simulink model "mvc_model_L"  (R2019a)
settings: Solver=FixedStepAuto  StartTime=0.0  StopTime=500  FixedStep=Ts  RelTol=1e-3  EnableMultiTasking=on
values from neighbouring files (symbols this model uses):
  f1_off_L = 0    [msstudy.m]
  f2_off_L = 0    [msstudy.m]
  f3_off_L = 0    [msstudy.m]
  f4_off_L = 0    [msstudy.m]
  f5_off_L = 0    [msstudy.m]
  f6_off_L = 0    [msstudy.m]
  maxtorquediff = 50    [msstudy.m]
  off_TA = 0    [msstudy.m]    (also in mvc_reflex.m = nanmean(tsmovavg(Input3.data(1:20000,1),'s',1000,1)))
  TA_MVC = 1    [msstudy.m]    (also in mvc_reflex.m = max((tsmovavg(abs(Input3.data(:,1)-off_TA),'s',1000,1))))
  Ts = 0.0005    [msstudy.m]
  tweight = 50*0.01*weight    [msstudy.m]    (also in weightcalc.m = weight/2)
undefined symbols (not defined in the file or in its folder): Pull, up
libraries: speedgoatlib_IO183 x6, powerlib_meascontrol x3, slrtlib x2
settings Model: Creator=vnalam  LastModifiedBy=vnalam
settings DataIOCC: LimitDataPoints=on  SaveFormat=StructureWithTime  ReturnWorkspaceOutputs=off
settings OptimizationCC: BlockReduction=off  OptimizeBlockIOStorage=off  BufferReuse=off  GlobalBufferReuse=off  ExpressionFolding=off  LocalBlockOutputs=off  LifeSpan=inf  OptimizeDataStoreBuffers=off  BusAssignmentInplaceUpdate=off
settings DebuggingCC: AllowSymbolicDim=off  SFUnexpectedBacktrackingDiag=warning  SFNoUnconditionalDefaultTransitionDiag=warning  SFExecutionAtInitializationDiag=none  ArithmeticOperatorsInVariantConditions=warning
settings HardwareCC: ProdBitPerPointer=32  ProdBitPerSizeT=32  ProdBitPerPtrDiffT=32  ProdLargestAtomicFloat=None  ProdWordSize=32  ProdLongLongMode=on  ProdHWDeviceType=Generic->32-bit x86 compatible
settings ModelReferenceCC: PropagateSignalLabelsOutOfModel=off
settings SFSimCC: SimUseLocalCustomCode=off
settings RTWCC: SystemTargetFile=slrt.tlc  TLCOptions=-axPCModelStackSizeKB=512  TemplateMakefile=slrt_default_tmf  Description=Simulink Real-Time  RTWUseLocalCustomCode=off  CodeExecutionProfiling=on  RTWCompilerOptimization=on
settings CodeAppCC: StateflowObjectComments=on
settings SimulinkRealTimeCC: PreserveStateflowLocalDataDimensions=off  xPCisDownloadable=off
settings ConfigComp: CovMetricSettings=dw  CovHtmlReporting=on  CovSaveCumulativeToWorkspaceVar=on  CovSaveSingleToWorkspaceVar=on  CovExternalEMLEnable=off

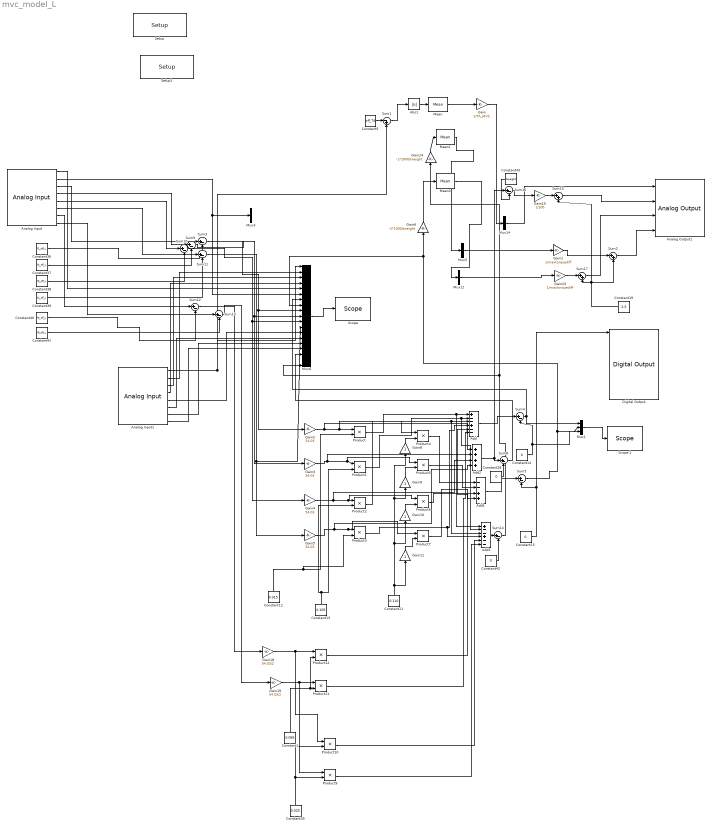
== system mvc_model_L ==
  Abs1 : Abs
  Add : Sum  Inputs=+--+--
  Add1 : Sum  Inputs=--++
  Add2 : Sum  Inputs=++++
  Add3 : Sum  Inputs=+--+--
  Analog Input : speedgoatlib_IO183/Analog Input  Priority=0  parModuleId=1  parSampTime=Ts  parPciSlot=-1  parAdChannelLow=1  parAdChannelHigh=8
      settings: SourceProductName=Simulink Real-Time: Speedgoat Library
  Analog Input1 : speedgoatlib_IO183/Analog Input  Priority=0  parModuleId=2  parSampTime=Ts  parPciSlot=-1  parAdChannelLow=1  parAdChannelHigh=8
      settings: SourceProductName=Simulink Real-Time: Speedgoat Library
  Analog Output1 : speedgoatlib_IO183/Analog Output  parModuleId=2  parSampTime=-1  parDaSimult=on  parPciSlot=-1  parDaChannels=[1 2 3 4]  parDaInit=[0 0 0 0]  parDaReset=[0 0 0 0]
      settings: SourceProductName=Simulink Real-Time: Speedgoat Library
  Constant1 : Constant  Value=0.095  SampleTime=-1
  Constant11 : Constant  Value=0.110  SampleTime=-1
  Constant12 : Constant  Value=0.315  SampleTime=-1
  Constant13 : Constant  Value=0.105  SampleTime=-1
  Constant{14..15,28,42} (4 alike) : Constant  Value=0  SampleTime=Ts
  Constant19 : Constant  Value=2.5  SampleTime=Ts
  Constant35 : Constant  Value=0.025  SampleTime=-1
  Constant36 : Constant  Value=f1_off_L  SampleTime=Ts
  Constant37 : Constant  Value=f2_off_L  SampleTime=Ts
  Constant38 : Constant  Value=f3_off_L  SampleTime=Ts
  Constant39 : Constant  Value=f4_off_L  SampleTime=Ts
  Constant40 : Constant  Value=f5_off_L  SampleTime=Ts
  Constant41 : Constant  Value=f6_off_L  SampleTime=Ts
  Constant43 : Constant  Value=tweight  SampleTime=Ts
  Constant5 : Constant  Value=off_TA  SampleTime=Ts
  Digital Output : speedgoatlib_IO183/Digital Output  parModuleId=2  parSampTime=Ts  parPciSlot=-1  parDoChannels=[1 2 3 4 5 6 7 8]  parDoInit=[0 0 0 0 0 0 0 0]  parDoReset=[1 1 1 1 1 1 1 1]
      settings: SourceProductName=Simulink Real-Time: Speedgoat Library
  Gain : Gain  Gain=1/TA_MVC
  Gain1 : Gain  Gain=1/maxtorquediff
  Gain{8..11} (4 alike) : Gain
  Gain14 : Gain  Gain=-1*1000/tweight
  Gain15 : Gain  Gain=1/100
  Gain18 : Gain  Gain=54.03/2
  Gain19 : Gain  Gain=54.03/2
  Gain{2..5} (4 alike) : Gain  Gain=54.03
  Gain23 : Gain  Gain=1/maxtorquediff
  Gain6 : Gain  Gain=-1*1000/tweight
  Mean : powerlib_meascontrol/Measurements/Mean  Freq=2  Vinit=0  Ts=0
      settings: SourceProductName=Simscape Electrical
  Mean1 : powerlib_meascontrol/Measurements/Mean  Freq=2  Vinit=0  Ts=0
      settings: SourceProductName=Simscape Electrical
  Mean2 : powerlib_meascontrol/Measurements/Mean  Freq=2  Vinit=0  Ts=0
      settings: SourceProductName=Simscape Electrical
  Mux1 : Mux  Inputs=3
  Mux{3,5,11,14} (4 alike) : Mux  Inputs=1
  Mux6 : Mux  Inputs=19
  Product{,1..7,9..12} (12 alike) : Product
  "Scope " : slrtlib/Displays and Logging/Scope   scopeno=3  scopetype=File  autostart=on  viewmode=Graphical redraw  formatstr='%15.6f'  grid=on  ylimits=[0,0]  nosamples=800000  noprepostsamples=0  interleave=1  triggermode=FreeRun  triggersignal=1  trigsignalfromport=off  triggerlevel=0.0  triggerslope=Either  triggerscope=1  triggersample=0  filename=MVC_L.dat  mode=Commit  writesize=512  autorestart=off  dynamicfilemode=off  maxwritefilesize=512*1024^2
  Scope 1 : slrtlib/Displays and Logging/Scope   scopeno=1  scopetype=Target  autostart=on  viewmode=Graphical sliding  formatstr='%15.6f'  grid=on  ylimits=[0,0]  nosamples=40000  noprepostsamples=0  interleave=1  triggermode=FreeRun  triggersignal=1  trigsignalfromport=off  triggerlevel=0.0  triggerslope=Either  triggerscope=1  triggersample=0  filename=data.dat  mode=Lazy  writesize=512  autorestart=off  dynamicfilemode=off  maxwritefilesize=512*1024^2
  Setup : speedgoatlib_IO183/Setup  parModuleId=1  parPciSlot=-1  parDaSimult=on  parAdCoupling=Single Ended  parAdRange=+-10V  parAdChannelLow=1  parAdChannelHigh=8  parDaChannels=[1:4]  parDaRange=0..5V  parDaInit=[0]  parDaReset=[0]  parDoChannels=[1:8]  parDoInit=[0]  parDoReset=[1]  parDiChannels=[9:16]  parIOPullReferenceFront=Pull-up (3.3V)  parIOPullReferenceRear=Pull-up (3.3V)
      settings: SourceProductName=Simulink Real-Time: Speedgoat Library
  Setup1 : speedgoatlib_IO183/Setup  parModuleId=2  parPciSlot=-1  parDaSimult=on  parAdCoupling=Single Ended  parAdRange=+-10V  parAdChannelLow=1  parAdChannelHigh=8  parDaChannels=[1:4]  parDaRange=0..5V  parDaInit=[0]  parDaReset=[0]  parDoChannels=[1:8]  parDoInit=[0]  parDoReset=[1]  parDiChannels=[9:16]  parIOPullReferenceFront=Pull-up (3.3V)  parIOPullReferenceRear=Pull-up (3.3V)
      settings: SourceProductName=Simulink Real-Time: Speedgoat Library
  Sum1 : Sum  Inputs=|-+
  Sum{3..5,8..14,16} (11 alike) : Sum  Inputs=|+-
  Sum15 : Sum  Inputs=|++
  Sum17 : Sum  Inputs=|++
  Sum2 : Sum  Inputs=|++
  wires:
  Constant5/1 -> Sum1/1
  Mean/1 -> Gain/1
  Sum1/1 -> Abs1/1
  Abs1/1 -> Mean/1
  Gain2/1 -> Add2/1, Product4/1, Product/1
  Gain3/1 -> Add2/2, Product5/1, Product1/1
  Gain4/1 -> Add2/3, Product6/1, Product2/1
  Gain5/1 -> Add2/4, Product7/1, Product3/1
  Constant11/1 -> Gain8/1, Gain9/1, Gain10/1, Gain11/1
  Gain8/1 -> Product4/2
  Gain9/1 -> Product5/2
  Gain10/1 -> Product6/2
  Gain11/1 -> Product7/2
  Product/1 -> Add3/1, Add/1
  Product1/1 -> Add3/2, Add/2
  Product2/1 -> Add3/3, Add/3
  Product3/1 -> Add3/4, Add/4
  Product4/1 -> Add1/1
  Product6/1 -> Add1/3
  Product5/1 -> Add1/2
  Product7/1 -> Add1/4
  Constant13/1 -> Product2/2, Product1/2
  Constant12/1 -> Product3/2, Product/2
  Constant14/1 -> Mux1/3, Sum4/2
  Constant15/1 -> Digital Output/1, Sum5/2
  Add/1 -> Sum4/1
  Add1/1 -> Sum5/1
  Mean1/1 -> Mux5/1
  Mux5/1 -> Gain1/1
  Gain1/1 -> Sum2/1
  Sum2/1 -> Analog Output1/4
  Constant19/1 -> Sum17/2, Sum15/2, Sum2/2
  Mean2/1 -> Mux11/1
  Mux11/1 -> Gain23/1
  Gain14/1 -> Mean1/1
  Gain6/1 -> Mean2/1
  Gain/1 -> Mux14/1
  Sum9/1 -> Mux6/10, Gain3/1
  Sum10/1 -> Mux6/11, Gain4/1
  Sum11/1 -> Mux6/12, Gain5/1
  Constant1/1 -> Product12/2, Product11/2
  Gain18/1 -> Product10/1, Product12/1
  Gain19/1 -> Product9/1, Product11/1
  Product12/1 -> Add/5
  Product11/1 -> Add/6
  Sum12/1 -> Gain18/1
  Sum13/1 -> Gain19/1
  Sum3/1 -> Mux6/9, Gain2/1
  Analog Input1/1 -> Mux6/1, Sum1/2
  Constant28/1 -> Sum8/2
  Add2/1 -> Sum8/1, Sum16/1
  Constant35/1 -> Product10/2, Product9/2
  Product10/1 -> Add3/5
  Product9/1 -> Add3/6
  Analog Input/3 -> Sum3/1
  Analog Input/5 -> Sum10/1
  Analog Input/4 -> Sum9/1
  Analog Input/6 -> Sum11/1
  Constant36/1 -> Sum3/2
  Constant37/1 -> Sum9/2
  Constant38/1 -> Sum10/2
  Constant39/1 -> Sum11/2
  Analog Input/7 -> Sum12/1
  Constant40/1 -> Sum12/2
  Analog Input/8 -> Sum13/1
  Constant41/1 -> Sum13/2
  Add3/1 -> Sum14/1
  Constant42/1 -> Sum14/2
  Sum14/1 -> Mux6/19, Gain14/1
  Gain15/1 -> Sum15/1
  Constant43/1 -> Sum16/2
  Sum16/1 -> Gain15/1
  Mux14/1 -> Analog Output1/1
  Sum15/1 -> Analog Output1/2
  Analog Input/1 -> Mux6/5
  Gain23/1 -> Sum17/1
  Sum17/1 -> Analog Output1/3
  Mux6/1 -> "Scope "/1
  Analog Input1/2 -> Mux6/2
  Analog Input1/3 -> Mux6/3
  Analog Input1/4 -> Mux6/4
  Analog Input/2 -> Mux3/1, Mux6/6
  Sum4/1 -> Mux6/7, Mux1/1
  Analog Input1/5 -> Mux6/13
  Analog Input1/6 -> Mux6/14
  Analog Input1/7 -> Mux6/15
  Analog Input1/8 -> Mux6/16
  Sum8/1 -> Mux6/17
  Mux1/1 -> Scope 1/1
  Sum5/1 -> Mux1/2, Mux6/8, Gain6/1
